simulink model "GSFR_Individual_Vars"  (R2019b)
settings: Solver=VariableStepAuto  StartTime=0  StopTime=20.0  MaxStep=0.01  RelTol=1e-3
model workspace (MAT data in the model file):
  H = [8 1]
values from neighbouring files (symbols this model uses):
  c = (((2*H*R)+(((D*R)+(K*Fh))*Tr))/(2*(D*R+K)))*wn    [Injections_plot.m]    (also in Monte_Carlo_GSFR_Half_Length_Injection.m; Monte_Carlo_GSFR_Ideal_Injection.m; Monte_Carlo_GSFR_Simplified_Injection.m; dpt_from_dft_H.m)
  D = 1.0    (= 1)    [Injections_plot.m]    (also in Monte_Carlo_GSFR_Half_Length_Injection.m; Monte_Carlo_GSFR_Ideal_Injection.m; Monte_Carlo_GSFR_Simplified_Injection.m; dpt_from_dft_H.m)
  K = 0.95    [Injections_plot.m]    (also in Monte_Carlo_GSFR_Half_Length_Injection.m; Monte_Carlo_GSFR_Ideal_Injection.m; Monte_Carlo_GSFR_Simplified_Injection.m; dpt_from_dft_H.m)
  Pd = -0.3    [Injections_plot.m]    (also in Monte_Carlo_GSFR_Half_Length_Injection.m; Monte_Carlo_GSFR_Ideal_Injection.m; Monte_Carlo_GSFR_Simplified_Injection.m; dpt_from_dft_H.m)
  R = 0.075    [Injections_plot.m]    (also in Monte_Carlo_GSFR_Half_Length_Injection.m = (0.05/3)*randn()+0.075; Monte_Carlo_GSFR_Ideal_Injection.m = (0.05/3)*randn()+0.075; Monte_Carlo_GSFR_Simplified_Injection.m = (0.05/3)*randn()+0.075; dpt_from_dft_H.m = 0.05)
  Tr = 9.0    (= 9)    [Injections_plot.m]    (also in Monte_Carlo_GSFR_Half_Length_Injection.m = 0.67*randn()+9; Monte_Carlo_GSFR_Ideal_Injection.m = 0.67*randn()+9; Monte_Carlo_GSFR_Simplified_Injection.m = 0.67*randn()+9; dpt_from_dft_H.m = 8)
  wn = sqrt((D*R+K)/(2*H*R*Tr))    [Injections_plot.m]    (also in Monte_Carlo_GSFR_Half_Length_Injection.m; Monte_Carlo_GSFR_Ideal_Injection.m; Monte_Carlo_GSFR_Simplified_Injection.m; dpt_from_dft_H.m)
settings Model: EnablePacing=on  PacingRate=1000  ParameterArgumentNames=H  OrderedModelArguments=off  Creator=ruiva  LastModifiedBy=ruiva

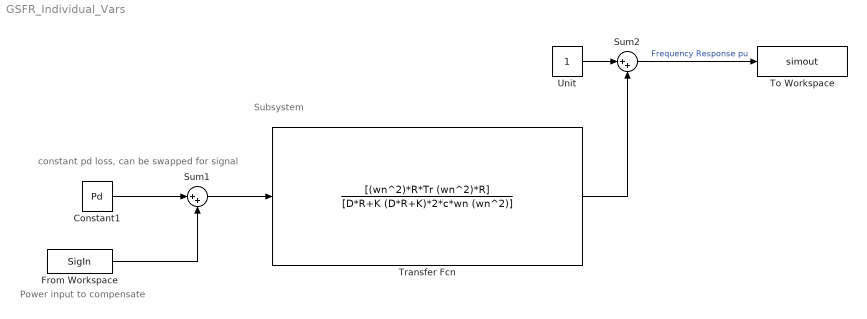
== system GSFR_Individual_Vars ==
  note: Subsystem
  note: Power input to compensate
  note: constant pd loss, can be swapped for signal
  Constant1 : Constant  Value=Pd
  From Workspace : FromWorkspace  VariableName=SigIn  SampleTime=0
  Sum1 : Sum  Inputs=|++
  Sum2 : Sum  Inputs=|++
  To Workspace : ToWorkspace  VariableName=simout  SaveFormat=Timeseries  SampleTime=-1
  Transfer Fcn : TransferFcn  Numerator=[(wn^2)*R*Tr (wn^2)*R]  Denominator=[D*R+K (D*R+K)*2*c*wn (wn^2)]
  Unit : Constant
  wires:
  Transfer Fcn/1 -> Sum2/2
  Unit/1 -> Sum2/1
  Sum2/1 -> To Workspace/1  "Frequency Response pu"
  From Workspace/1 -> Sum1/2
  Sum1/1 -> Transfer Fcn/1
  Constant1/1 -> Sum1/1
